simulink model "metron"  (R2019b)
settings: Solver=VariableStepAuto  StartTime=0.0  StopTime=10.0  RelTol=1e-3
values from neighbouring files (symbols this model uses):
  c = set_controller()    [lab3.m]    (also in metronomo.m)
  s = rmfield(s, 'm')    [getWnfromSimulation.m]    (also in lab3.m = set_system9(l_ls(2),m); lgetNLS.m = set_system9(new_l(j,i),s.m); metronomo.m = set_system9(l_ls(2),m))
settings Model: Creator=joaotiagoalmeida  LastModifiedBy=joaotiagoalmeida

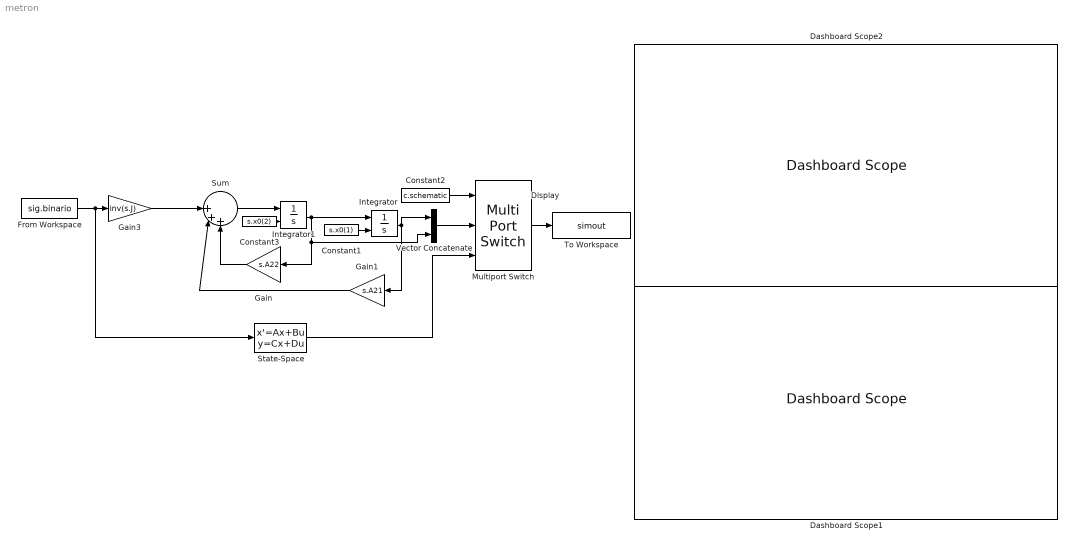
== system metron ==
  Constant1 : Constant  Value=s.x0(1)  SampleTime=c.samptime
  Constant2 : Constant  Value=c.schematic  SampleTime=c.samptime
  Constant3 : Constant  Value=s.x0(2)  SampleTime=c.samptime
  Dashboard Scope1 : DashboardScope
  Dashboard Scope2 : DashboardScope
  Display : DisplayBlock  LabelPosition=Hide  Format=short  Transparency=1
  From Workspace : FromWorkspace  VariableName=sig.binario  SampleTime=c.samptime
  Gain : Gain  Gain=s.A22
  Gain1 : Gain  Gain=s.A21
  Gain3 : Gain  Gain=inv(s.J)
  Integrator : Integrator  InitialConditionSource=external
  Integrator1 : Integrator  InitialConditionSource=external  IgnoreLimit=on  ZeroCross=off
  Multiport Switch : MultiPortSwitch  DataPortOrder=Specify indices  DataPortIndices={5,[6]}
  State-Space : StateSpace  A=s.sys.A  B=s.sys.B  C=s.sys.C  D=s.sys.D  InitialCondition=s.x0
  Sum : Sum  Inputs=||+++
  To Workspace : ToWorkspace  VariableName=simout  SaveFormat=Timeseries  SampleTime=c.samptime
  Vector Concatenate : Concatenate
  wires:
  Gain3/1 -> Sum/1
  Sum/1 -> Integrator1/1
  Integrator1/1 -> Integrator/1, Vector Concatenate/2, Gain/1
  Multiport Switch/1 -> To Workspace/1
  Integrator/1 -> Vector Concatenate/1, Gain1/1
  Gain/1 -> Sum/3
  Gain1/1 -> Sum/2
  From Workspace/1 -> State-Space/1, Gain3/1
  State-Space/1 -> Multiport Switch/3
  Constant2/1 -> Multiport Switch/1
  Constant1/1 -> Integrator/2
  Vector Concatenate/1 -> Multiport Switch/2
  Constant3/1 -> Integrator1/2
